simulink model "x2_lidar_ros_toolbox"  (R2024b)
settings: Solver=FixedStepAuto  StartTime=0.0  StopTime=10  FixedStep=Ts  RelTol=1e-3
InitFcn:
  | Ts=0.01;
model workspace (MAT data in the model file):
  SL_ROS_VariableLengthArrays_MaxSizes.CommonInfo.ArrayTruncateAction = 'EmitWarning'
  SL_ROS_VariableLengthArrays_MaxSizes.MsgTypeMap = containers.Map
  SL_ROS_VariableLengthArrays_MaxSizes.MsgTypeMap.serialization.keys = {'sensor_msgs/LaserScan', 'std_msgs/Header'}
  SL_ROS_VariableLengthArrays_MaxSizes.MsgTypeMap.serialization.values{1}(1).PropertyName = 'intensities'
  SL_ROS_VariableLengthArrays_MaxSizes.MsgTypeMap.serialization.values{1}(1).DataType = 'single'
  SL_ROS_VariableLengthArrays_MaxSizes.MsgTypeMap.serialization.values{1}(1).MaxLength = 1
  SL_ROS_VariableLengthArrays_MaxSizes.MsgTypeMap.serialization.values{1}(2).PropertyName = 'ranges'
  SL_ROS_VariableLengthArrays_MaxSizes.MsgTypeMap.serialization.values{1}(2).DataType = 'single'
  SL_ROS_VariableLengthArrays_MaxSizes.MsgTypeMap.serialization.values{1}(2).MaxLength = 6
  SL_ROS_VariableLengthArrays_MaxSizes.MsgTypeMap.serialization.values{2}.PropertyName = 'frame_id'
  SL_ROS_VariableLengthArrays_MaxSizes.MsgTypeMap.serialization.values{2}.DataType = 'uint8'
  SL_ROS_VariableLengthArrays_MaxSizes.MsgTypeMap.serialization.values{2}.MaxLength = 11
  SL_ROS_VariableLengthArrays_MaxSizes.MsgTypeMap.serialization.uniformity = 0
  SL_ROS_VariableLengthArrays_MaxSizes.MsgTypeMap.serialization.keyType = 'char'
  SL_ROS_VariableLengthArrays_MaxSizes.MsgTypeMap.serialization.valueType = 'any'
undefined symbols (not defined in the file): angle_increment, angle_max, angle_min, header, intensities, intensities_SL_Info, range_max, range_min, ranges, ranges_SL_Info
libraries: ros2lib x3, instrumentseriallib x2
settings Model: Creator=System-10  LastModifiedBy=01149
settings DataIOCC: ExternalInput=AngleFSA
settings OptimizationCC: EnhancedBackFolding=on  PassReuseOutputArgsAs=Individual arguments  ZeroExternalMemoryAtStartup=off  ZeroInternalMemoryAtStartup=off  MaxStackSize=64  OptimizeBlockOrder=speed  DifferentSizesBufferReuse=on  OptimizationCustomize=off  EfficientTunableParamExpr=on
settings DebuggingCC: ParameterTunabilityLossMsg=error
settings HardwareCC: TargetBitPerPointer=64  TargetBitPerSizeT=64  TargetBitPerPtrDiffT=64  TargetLargestAtomicFloat=Float  TargetIntDivRoundTo=Zero  TargetEndianess=LittleEndian  TargetWordSize=64  TargetHWDeviceType=Intel->x86-64 (Windows64)
settings ModelReferenceCC: PropagateVarSize=During execution
settings SFSimCC: SimTargetLang=C++
settings RTWCC: Description=Embedded Coder  SystemTargetFile=ert.tlc  HardwareBoard=Robot Operating System 2 (ROS 2)  TLCOptions="-aInlineSetEventsForThisBaseRateFcn=TLC_FALSE -aSuppressMultiTaskScheduler=TLC_FALSE  -aRateBasedStepFcn=0"  TemplateMakefile=ert_default_tmf  Toolchain=Colcon Tools  TargetLang=C++  GPUComputeCapability=3.5
settings CodeAppCC: ForceParamTrailComments=on  IgnoreCustomStorageClasses=off  OperatorAnnotations=on  SimulinkDataObjDesc=on  SFDataObjDesc=on  InsertBlockDesc=on
settings ERTTargetCC: CodeInterfacePackaging=C++ class  SupportVariableSizeSignals=on  InlinedParameterPlacement=Hierarchical  RootIOFormat=Structure reference  DynamicArrayContainerType=coder::array

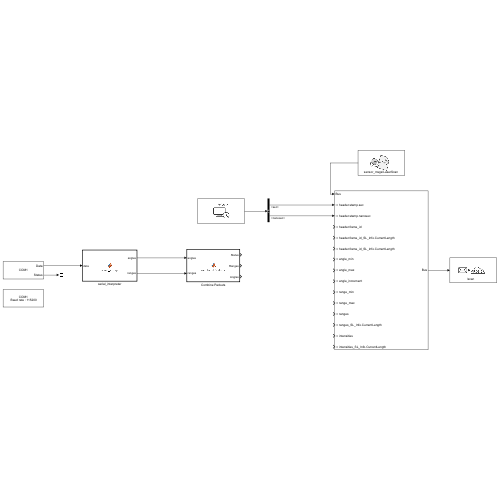
[thumbnail: Simulink's stored preview of the top-level diagram]
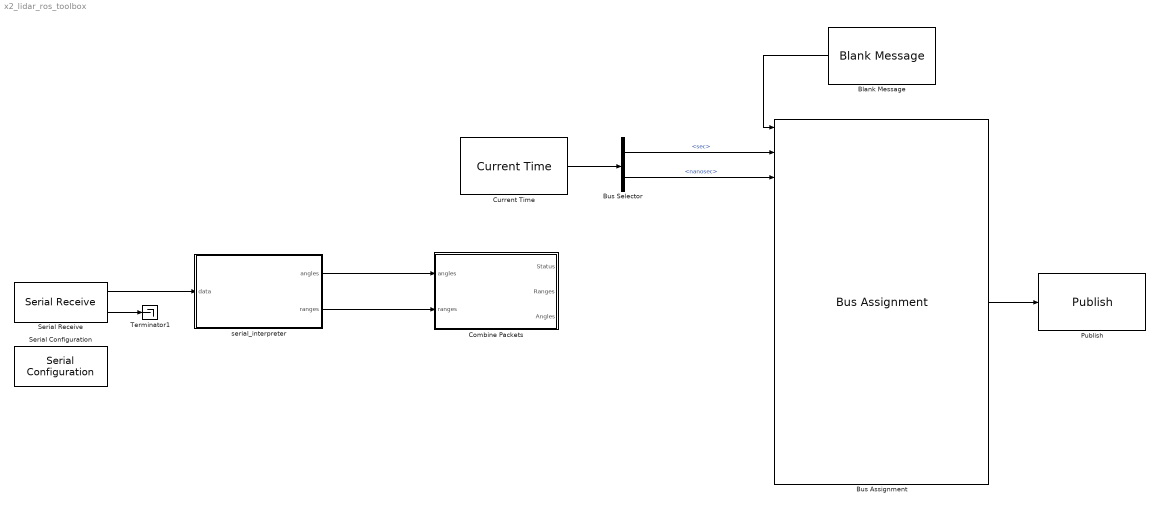
== system x2_lidar_ros_toolbox ==
  Blank Message : ros2lib/Blank Message  messageClass=Message  entityType=sensor_msgs/LaserScan  messageType=sensor_msgs/LaserScan  SampleTime=Ts
      settings: LibrarySourceBlock=roslib/ROS 2/Blank Message
  Bus Assignment : BusAssignment  AssignedSignals=header.stamp.sec,header.stamp.nanosec,header.frame_id,header.frame_id_SL_Info.CurrentLength,header.frame_id_SL_Info.CurrentLength,angle_min,angle_max,angle_increment,range_min,range_max,ranges,ranges_SL_Info.CurrentLength,intensities,intensities_SL_Info.CurrentLength
  Bus Selector : BusSelector  OutputSignals=sec,nanosec
  Combine Packets : MATLAB Function  TreatAsAtomicUnit=on
  Current Time : ros2lib/Current Time  OutputFormat=bus  SampleTime=-1  ModelName=Lidar
      settings: LibrarySourceBlock=roslib/ROS 2/Current Time
  Publish : ros2lib/Publish  topicSource=Specify your own  topic=/scan  messageType=sensor_msgs/LaserScan  QOSHistory=Keep last  QOSDepth=1  QOSReliability=Reliable  QOSDurability=Volatile  QOSDeadline=Inf  QOSLifespan=Inf  QOSLiveliness=Automatic  QOSLeaseDuration=Inf  QOSAvoidROSNamespaceConventions=off
      settings: LibrarySourceBlock=roslib/ROS 2/Publish
  Serial Configuration : instrumentseriallib/Serial Configuration  Priority=-200000  PortSel=COM1  Port=COM1  ComPort=COM1  BaudRate=115200  DataBits=8  Parity=none  StopBits=1  ByteOrder=little-endian  FlowControl=none  Timeout=10  SimulateUsing=Interpreted execution  BlockInModel=on  aMode=1
  Serial Receive : instrumentseriallib/Serial Receive  Priority=1  PortSel=COM1  Port=COM1  ComPort=COM1  DataType=uint8  SaveDataType=uint8  ToggleHeader=off  Header=[170 85]  ToggleDataSize=on  DataSize=[1 2000]  ToggleTerminator=off  Terminator=<none>  CustomTerminator=[]  InputFormat=Column major  EnableBlockingMode=off  ActionDataUnavailable=Output last received value  ActionWhenDataUnavailable=Output last received value  CustomValue=111  SampleTime=Ts  SimulateUsing=Interpreted execution  BlockInModel=on  aMode=1
  Terminator1 : Terminator
  serial_interpreter : MATLAB Function  TreatAsAtomicUnit=on
  wires:
  Blank Message/1 -> Bus Assignment/1
  Current Time/1 -> Bus Selector/1
  Bus Assignment/1 -> Publish/1
  serial_interpreter/1(angles) -> Combine Packets/1(angles)
  serial_interpreter/2(ranges) -> Combine Packets/2(ranges)
  Serial Receive/2 -> Terminator1/1
  Serial Receive/1 -> serial_interpreter/1(data)
  Bus Selector/1 -> Bus Assignment/2  "<sec>"
  Bus Selector/2 -> Bus Assignment/3  "<nanosec>"

== matlab function x2_lidar_ros_toolbox/Combine Packets ==
  settings: updateMethod=DISCRETE  sampleTime=Ts
  data: Status output boolean; Ranges output size=[1 400]; angles input; Angles output size=[1 400]; ranges input
function [Status,Ranges,Angles]  = combinePackets(angles,ranges)
    persistent count; 
    persistent elemAngles;
    persistent elemRanges;
    
    if sum(angles) == 0
        Angles = zeros(1,400);
        Ranges = zeros(1,400);
        Status = boolean(0);
        return;
    end

    if isempty(count)
        count = 0;
        elemAngles = zeros(1,400);
        elemRanges = zeros(1,400);
    end
        
    for i = 1:length(angles)
        elemAngles(i+count) = angles(i);
        elemRanges(i+count) = ranges(i);
    end
    if count < (length(elemAngles)-length(angles))
        count = count + length(angles);
        Angles = zeros(1,400);
        Ranges = zeros(1,400);
        Status = boolean(0);
    else
        count = 0;
        %Current Angles as 1x400 array [rad].
        Angles = deg2rad(elemAngles);
        %Current Ranges as 1x400 array [meter].
        Ranges = elemRanges;
        Status = boolean(1);
    end
end

== matlab function x2_lidar_ros_toolbox/serial_interpreter ==
  settings: updateMethod=DISCRETE  sampleTime=Ts
  data: data input; angles output; ranges output
function [angles,ranges] = serial_interp(data)

    persistent lastData;
    persistent indices;
    persistent currentIdx;
    persistent Si;
    persistent AngleSi;

    if isempty(lastData)
        lastData = uint8(zeros(1,size(data,2)));
        Si = zeros(1, 40);
        AngleSi = zeros(1, 40);
    end
    if isempty(indices) || ~isequal(data, lastData)
        indices = find(data==170 | data==85);
        indices = indices(diff(indices) == 1);
        indices = indices(diff(indices) == 90);
        currentIdx = 1;
        lastData = data;
    end

    if currentIdx <= numel(indices)
         FSA = double(bitshift ...
             (double ...
             (bitor ...
             (bitshift ...
             (uint16(data(1, indices(currentIdx)+5)), 8), uint16(data(1, indices(currentIdx)+4) ...
             ), ...
             'uint16')), ...
             -1) / 64);
         LSA = double(bitshift ...
             (double ...
             (bitor ...
             (bitshift ...
             (uint16(data(1, indices(currentIdx)+7)), 8), uint16(data(1, indices(currentIdx)+6) ...
             ), ...
             'uint16')), ...
             -1) / 64);
         
         diffAngle = mod((LSA - FSA),360);

         for j = 1:80
             if mod(j, 2) == 0
                Si(j / 2) = double(bitor ...
                    (bitshift ...
                    (uint16(data(1, (indices(currentIdx)+9)+j)), 8), ...
                    uint16(data(1, (indices(currentIdx)+9)+j-1)), 'uint16') ...
                    );
                if Si(j / 2) == 0
                    AngleSi(j / 2) = ((diffAngle / (40 - 1)) * ((j / 2) - 1) + FSA);
                else
                    AngleSi(j / 2) = ((diffAngle / (40 - 1)) * ((j / 2) - 1) + FSA) + atan(21.8*((155.3-Si((j / 2)))/(155.3*Si((j / 2)))));
                end
             end
         end
        %Current Angles as 1x40 array [deg].
        angles = AngleSi;
    
        %Current Ranges as 1x40 array [meter].
        ranges = Si / 4000;
        currentIdx = currentIdx + 1;
    else
        angles = zeros(1, 40);
        ranges = zeros(1, 40);
    end
end
